simulink model "voltage_inverter"  (R2023a)
settings: Solver=VariableStepAuto  StartTime=0.0  StopTime=0.2  RelTol=1e-3
undefined symbols (not defined in the file): frequency, fsw, kpi, kpv, krv, omega, vc_c, vc_l, vdc, vref_rms
libraries: spsGroundLib x3, spsHalfBridgeConverterLib x3, spsThreePhaseParallelRLCBranchLib x3, spsThreePhaseVIMeasurementLib x3, spsabctoAlphaBetaZeroLib x3, spsAlphaBetaZerotoabcLib x1, spsDCVoltageSourceLib x1, eePwmGeneratorTwoLevel x1, spsThreePhaseProgrammableVoltageSourceLib x1, spspowerguiLib x1
settings Model: Creator=MrSam  LastModifiedBy=15185

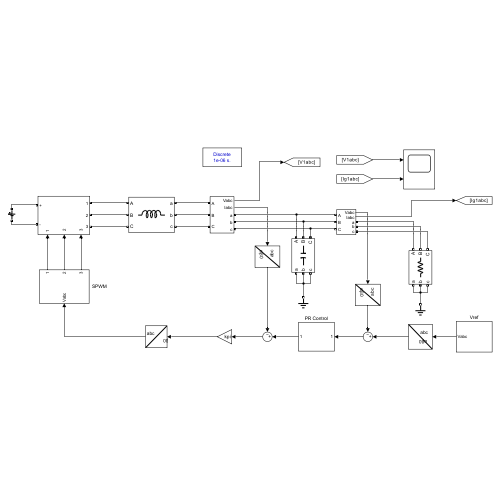
[thumbnail: Simulink's stored preview of the top-level diagram]
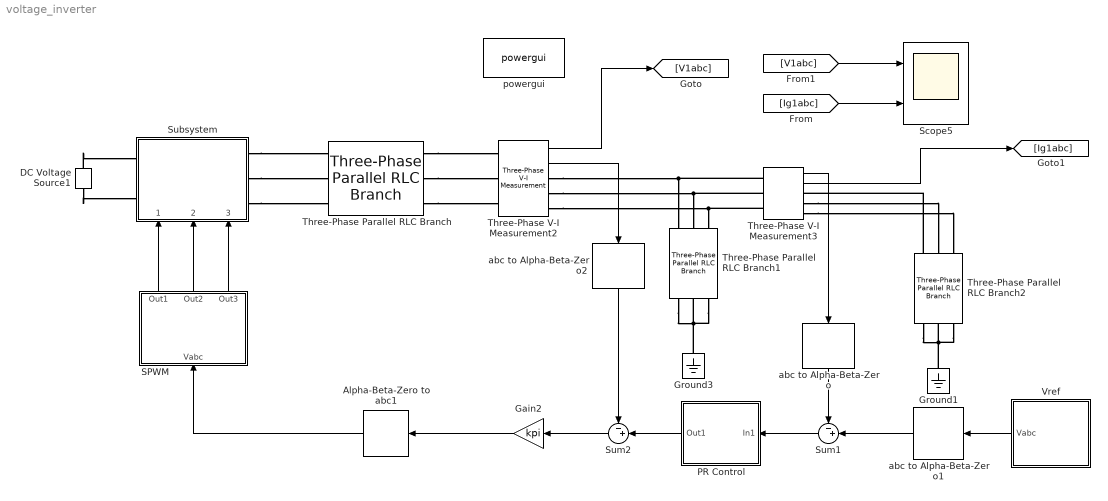
== system voltage_inverter ==
  Alpha-Beta-Zero to abc1 : spsAlphaBetaZerotoabcLib/Alpha-Beta-Zero to abc
      settings: LibrarySourceBlock=|
      | sps_lib/Control/Alpha-Beta-Zero
      | to abc
  DC Voltage Source1 : spsDCVoltageSourceLib/DC Voltage Source  Amplitude=vdc  Measurements=None
  Gain2 : Gain  Gain=kpi
  Ground1 : spsGroundLib/Ground  LConnTagsString=a
  Ground3 : spsGroundLib/Ground  LConnTagsString=a
  PR Control : Subsystem
  SPWM : Subsystem
  Scope5 : Scope  NumInputPorts=2
  Subsystem : Subsystem
      settings: PortSchema="{\"entries\":[{\"content\":{\"sides\":[{\"content\":{\"connectorIds\":[\"LConn1\",\"LConn2\"]},\"type\":\"ConnectorPlacement.EquallySpacedRectSide\",\"uuid\":\"21765539-0567-4900-b052-fb0c809e49e6\"},{\"content\":{\"connectorIds\":[\"RConn1\",\"RConn2\",\"RConn3\"],\"side\":\"RIGHT\"},\"type\":\"ConnectorPlacement.EquallySpacedRectSide\",\"uuid\":\"da60e673-aefd-4ef6-b5b1-e42a137712f7\"},{\"content\":{\"side\":\"TOP\"},\"type\":\"ConnectorPlacement.EquallySpacedRectSide\",\"uuid\":\"b6e664be-1a8c-4c9c-bd73-b93bd6e53381\"},{\"content\":{\"connectorIds\":[\"In1\",\"In2\",\"In3\"],\"side\":\"BOTTOM\"},\"type\":\"ConnectorPlacement.EquallySpacedRectSide\",\"uuid\":\"f785bed7-33ce-41e0-9620-ddd9724794f7\"}]},\"type\":\"ConnectorPlacement.EquallySpacedConnector\",\"uuid\":\"3eaff965-cae1-44ee-8f3f-ae8df46f200b\"}],\"packageUris\":[\"http://schema.mathworks.com/mf0/Connector/R2020b\"],\"version\":\"1.0\"}"
  Sum1 : Sum  Inputs=-+|
  Sum2 : Sum  Inputs=-+|
  Three-Phase Parallel RLC Branch : spsThreePhaseParallelRLCBranchLib/Three-Phase Parallel RLC Branch  LConnTagsString=A|B|C  RConnTagsString=A|B|C  BranchType=L  Resistance=1  Inductance=vc_l/(2*pi*frequency)  Capacitance=1e-6  Measurements=None
  Three-Phase Parallel RLC Branch1 : spsThreePhaseParallelRLCBranchLib/Three-Phase Parallel RLC Branch  LConnTagsString=A|B|C  RConnTagsString=A|B|C  BranchType=C  Resistance=1  Inductance=vc_l  Capacitance=1/(vc_c*2*pi*frequency)  Measurements=None
  Three-Phase Parallel RLC Branch2 : spsThreePhaseParallelRLCBranchLib/Three-Phase Parallel RLC Branch  LConnTagsString=A|B|C  RConnTagsString=A|B|C  BranchType=R  Resistance=10  Inductance=1e-3  Capacitance=1e-6  Measurements=None
  Three-Phase V-I Measurement2 : spsThreePhaseVIMeasurementLib/Three-Phase V-I Measurement  VoltageMeasurement=phase-to-ground  SetLabelV=off  LabelV=Vabc  Vpu=off  VpuLL=off  CurrentMeasurement=yes  SetLabelI=off  LabelI=Iabc  Ipu=off  Pbase=100e6  Vbase=500e3  OutputType=Complex  PhasorSimulation=off  PSBequivalent=0
  Three-Phase V-I Measurement3 : spsThreePhaseVIMeasurementLib/Three-Phase V-I Measurement  VoltageMeasurement=phase-to-ground  SetLabelV=off  LabelV=Vabc  Vpu=off  VpuLL=off  CurrentMeasurement=yes  SetLabelI=off  LabelI=Iabc  Ipu=off  Pbase=100e6  Vbase=500e3  OutputType=Complex  PhasorSimulation=off  PSBequivalent=0
  Vref : Subsystem
  abc to Alpha-Beta-Zero : spsabctoAlphaBetaZeroLib/abc to Alpha-Beta-Zero
  abc to Alpha-Beta-Zero1 : spsabctoAlphaBetaZeroLib/abc to Alpha-Beta-Zero
  abc to Alpha-Beta-Zero2 : spsabctoAlphaBetaZeroLib/abc to Alpha-Beta-Zero
  powergui : spspowerguiLib/powergui  Priority=1  SimulationMode=Discrete  SampleTime=1e-6  frequency=60  Iterations=50  frequencyindice=50  Pbase=100e6  ErrMax=1e-4  UnitsV=kV  UnitsW=MW  buscounter=0  FunctionMessages=off  echomessages=off  EnableUseOfTLC=off  CurrentSourceSwitches=off  DisableSnubberDevices=off  DisableRonSwitches=off  DisableVfSwitches=off  DisplayEquations=off  AutomaticDiscreteSolvers=off  SolverType=Tustin/Backward Euler (TBE)  Interpol=off  ExternalGateDelay=off  methode=off  Ts=100  x0status=blocks  SPID=on  SwTol=0  HookPort=off  NonlinearTolerance=1e-4  nMaxIteration=100  ContinueOnMaxIteration=off  RestoreLinks=warning  ResistiveCurrentMeasurement=off  Frange=[0:2:500]  Ylog=off  Xlog=on  ShowGrid=off  save=off  variable=ZData  structure=0  ZoomFFT=off  StartTime=0.0  cycles=1  DisplayStyle=1  fundamental=60  FreqAxis=off  MaxFrequency=1000  frequencyindicesteady=1  RmsSteady=1  display=off
  wires:
  Three-Phase V-I Measurement3/1 -> abc to Alpha-Beta-Zero/1
  abc to Alpha-Beta-Zero1/1 -> Sum1/2
  abc to Alpha-Beta-Zero/1 -> Sum1/1
  abc to Alpha-Beta-Zero2/1 -> Sum2/1
  Three-Phase V-I Measurement2/2 -> abc to Alpha-Beta-Zero2/1
  Sum2/1 -> Gain2/1
  Gain2/1 -> Alpha-Beta-Zero to abc1/1
  Sum1/1 -> PR Control/1(In1)
  PR Control/1(Out1) -> Sum2/2
  Vref/1(Vabc) -> abc to Alpha-Beta-Zero1/1
  Alpha-Beta-Zero to abc1/1 -> SPWM/1(Vabc)
  SPWM/1(Out1) -> Subsystem/1(" 1 ")
  SPWM/2(Out2) -> Subsystem/2("  2")
  SPWM/3(Out3) -> Subsystem/3("  3")
  Three-Phase V-I Measurement2/1 -> [V1abc]
  [Ig1abc] -> Scope5/2
  [V1abc] -> Scope5/1
  Three-Phase V-I Measurement3/2 -> [Ig1abc]
  connections:
  Three-Phase Parallel RLC Branch/RConn1 -- Three-Phase V-I Measurement2/LConn1
  Three-Phase Parallel RLC Branch/RConn2 -- Three-Phase V-I Measurement2/LConn2
  Three-Phase Parallel RLC Branch/RConn3 -- Three-Phase V-I Measurement2/LConn3
  Three-Phase V-I Measurement2/RConn1 -- Three-Phase Parallel RLC Branch1/LConn1 -- Three-Phase V-I Measurement3/LConn1
  Three-Phase V-I Measurement2/RConn2 -- Three-Phase V-I Measurement3/LConn2 -- Three-Phase Parallel RLC Branch1/LConn2
  Three-Phase V-I Measurement2/RConn3 -- Three-Phase Parallel RLC Branch1/LConn3 -- Three-Phase V-I Measurement3/LConn3
  Ground3/LConn1 -- Three-Phase Parallel RLC Branch1/RConn1 -- Three-Phase Parallel RLC Branch1/RConn3 -- Three-Phase Parallel RLC Branch1/RConn2
  Ground1/LConn1 -- Three-Phase Parallel RLC Branch2/RConn1 -- Three-Phase Parallel RLC Branch2/RConn3 -- Three-Phase Parallel RLC Branch2/RConn2
  DC Voltage Source1/RConn1 -- Subsystem/LConn1
  DC Voltage Source1/LConn1 -- Subsystem/LConn2
  Subsystem/RConn1 -- Three-Phase Parallel RLC Branch/LConn1
  Subsystem/RConn2 -- Three-Phase Parallel RLC Branch/LConn2
  Subsystem/RConn3 -- Three-Phase Parallel RLC Branch/LConn3
  Three-Phase V-I Measurement3/RConn3 -- Three-Phase Parallel RLC Branch2/LConn3
  Three-Phase Parallel RLC Branch2/LConn1 -- Three-Phase V-I Measurement3/RConn1
  Three-Phase V-I Measurement3/RConn2 -- Three-Phase Parallel RLC Branch2/LConn2

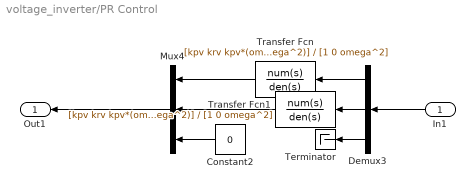
== system voltage_inverter/PR Control ==
  In1 : Inport
  Constant2 : Constant  Value=0
  Demux3 : Demux  Outputs=3
  Mux4 : Mux  Inputs=3
  Terminator : Terminator
  Transfer Fcn : TransferFcn  Numerator=[kpv krv kpv*(omega^2)]  Denominator=[1 0 omega^2]
  Transfer Fcn1 : TransferFcn  Numerator=[kpv krv kpv*(omega^2)]  Denominator=[1 0 omega^2]
  Out1 : Outport
  wires:
  Transfer Fcn/1 -> Mux4/1
  Mux4/1 -> Out1/1
  Demux3/1 -> Transfer Fcn/1
  Demux3/2 -> Transfer Fcn1/1
  Constant2/1 -> Mux4/3
  Transfer Fcn1/1 -> Mux4/2
  In1/1 -> Demux3/1
  Demux3/3 -> Terminator/1

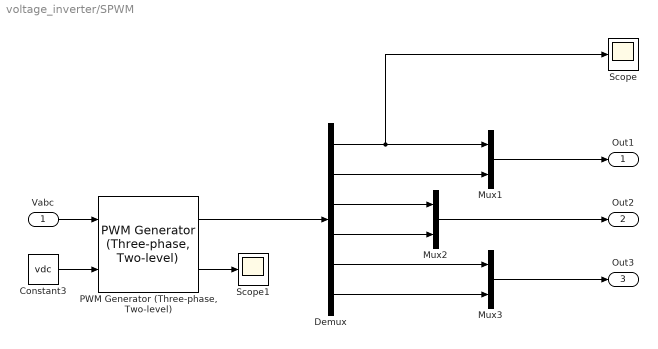
== system voltage_inverter/SPWM ==
  Vabc : Inport
  Constant3 : Constant  Value=vdc
  Demux : Demux  Outputs=6
  Mux1 : Mux  Inputs=2
  Mux2 : Mux  Inputs=2
  Mux3 : Mux  Inputs=2
  "PWM Generator (Three-phase, Two-level)" : eePwmGeneratorTwoLevel/PWM Generator (Three-phase, Two-level)  PWMMode=Continuous PWM (CPWM)  CPWMMode=SPWM: sinusoidal PWM  DPWMMode=60 DPWM: 60 degree discontinuous PWM  fsw=fsw  Ts=1/(60*fsw)
      settings: LibrarySourceBlock=|
      | ee_sl_lib/Pulse Width
      | Modulation/PWM Generator
      | (Three-phase, Two-level)
  Scope : Scope
  Scope1 : Scope
  Out1 : Outport
  Out2 : Outport  Port=2
  Out3 : Outport  Port=3
  wires:
  "PWM Generator (Three-phase, Two-level)"/2 -> Scope1/1
  Demux/2 -> Mux1/2
  Vabc/1 -> "PWM Generator (Three-phase, Two-level)"/1
  Demux/6 -> Mux3/2
  Demux/1 -> Scope/1, Mux1/1
  Constant3/1 -> "PWM Generator (Three-phase, Two-level)"/2
  Mux2/1 -> Out2/1
  Demux/4 -> Mux2/2
  "PWM Generator (Three-phase, Two-level)"/1 -> Demux/1
  Demux/3 -> Mux2/1
  Demux/5 -> Mux3/1
  Mux1/1 -> Out1/1
  Mux3/1 -> Out3/1

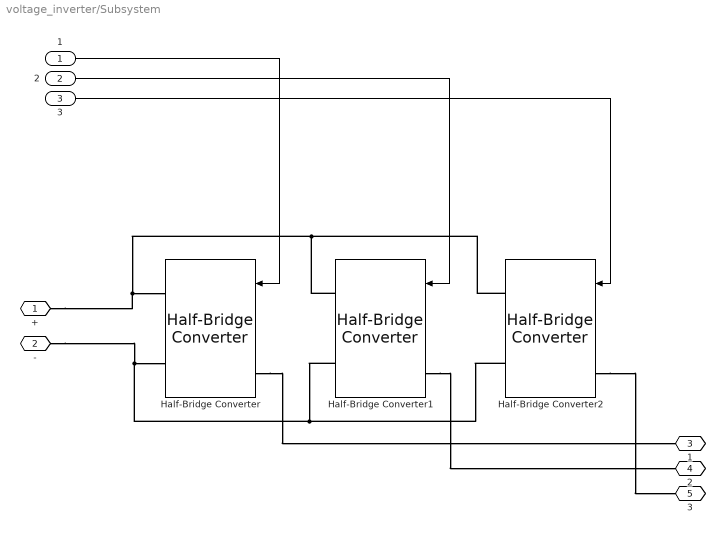
== system voltage_inverter/Subsystem ==
  " 1 " : Inport
  "  2" : Inport  Port=2
  "  3" : Inport  Port=3
  Half-Bridge Converter : spsHalfBridgeConverterLib/Half-Bridge Converter  ModelType=Switching devices  Ron=1e-3  Rs=1e6  Cs=inf  Vforward=[0,0]  Ron_Diode=1e-3  Rs_Diode=1e6  Cs_Diode=inf  Vf_Diode=1e-3  Rs_CurrentSource=inf  Ron_ACsource=1e-3
      settings: LibrarySourceBlock=sps_lib/Power Electronics/Half-Bridge Converter
  Half-Bridge Converter1 : spsHalfBridgeConverterLib/Half-Bridge Converter  ModelType=Switching devices  Ron=1e-3  Rs=1e6  Cs=inf  Vforward=[0,0]  Ron_Diode=1e-3  Rs_Diode=1e6  Cs_Diode=inf  Vf_Diode=1e-3  Rs_CurrentSource=inf  Ron_ACsource=1e-3
      settings: LibrarySourceBlock=sps_lib/Power Electronics/Half-Bridge Converter
  Half-Bridge Converter2 : spsHalfBridgeConverterLib/Half-Bridge Converter  ModelType=Switching devices  Ron=1e-3  Rs=1e6  Cs=inf  Vforward=[0,0]  Ron_Diode=1e-3  Rs_Diode=1e6  Cs_Diode=inf  Vf_Diode=1e-3  Rs_CurrentSource=inf  Ron_ACsource=1e-3
      settings: LibrarySourceBlock=sps_lib/Power Electronics/Half-Bridge Converter
  + : PMIOPort  Side=Left
  - : PMIOPort  Port=2  Side=Left
  1 : PMIOPort  Port=3  Side=Right
  2 : PMIOPort  Port=4  Side=Right
  3 : PMIOPort  Port=5  Side=Right
  wires:
  "  2"/1 -> Half-Bridge Converter1/1
  "  3"/1 -> Half-Bridge Converter2/1
  " 1 "/1 -> Half-Bridge Converter/1
  connections:
  Half-Bridge Converter/LConn1 -- 1/RConn1
  Half-Bridge Converter1/RConn1 -- Half-Bridge Converter2/RConn1 -- +/RConn1 -- Half-Bridge Converter/RConn1
  Half-Bridge Converter2/RConn2 -- Half-Bridge Converter1/RConn2 -- -/RConn1 -- Half-Bridge Converter/RConn2
  Half-Bridge Converter2/LConn1 -- 3/RConn1
  Half-Bridge Converter1/LConn1 -- 2/RConn1

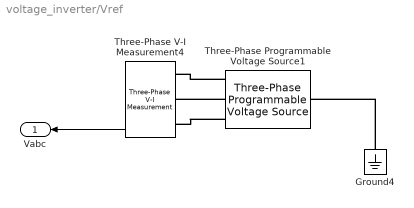
== system voltage_inverter/Vref ==
  Ground4 : spsGroundLib/Ground  LConnTagsString=a
  Three-Phase Programmable Voltage Source1 : spsThreePhaseProgrammableVoltageSourceLib/Three-Phase Programmable Voltage Source  PositiveSequence="[vref_rms  0 frequency]"  VariationEntity=None  VariationType=Table of time-amplitude pairs  VariationTypeAlt=Step  VariationStep=0.5  VariationRate=10  VariationMagnitude=0.3  VariationFrequency=2  VariationTiming=[1 2]  VariationPhaseA=off  Amplitudes=[1 0.8 1.2 1.0]  TimeValues=[0 0.1 0.15 0.2]  HarmonicGeneration=off  HarmonicA=[3 0.2 -25 0]  HarmonicB=[2 0.15 35 2]  Timing="[0.05  3]"  BusType=swing  Pref=0  Qref=0  Qmin=-inf  Qmax=inf
  Three-Phase V-I Measurement4 : spsThreePhaseVIMeasurementLib/Three-Phase V-I Measurement  VoltageMeasurement=phase-to-ground  SetLabelV=off  LabelV=Vabc  Vpu=off  VpuLL=off  CurrentMeasurement=yes  SetLabelI=off  LabelI=Iabc  Ipu=off  Pbase=100e6  Vbase=500e3  OutputType=Complex  PhasorSimulation=off  PSBequivalent=0
  Vabc : Outport
  wires:
  Three-Phase V-I Measurement4/1 -> Vabc/1
  connections:
  Three-Phase Programmable Voltage Source1/RConn2 -- Three-Phase V-I Measurement4/LConn2
  Three-Phase Programmable Voltage Source1/RConn3 -- Three-Phase V-I Measurement4/LConn3
  Three-Phase Programmable Voltage Source1/RConn1 -- Three-Phase V-I Measurement4/LConn1
  Ground4/LConn1 -- Three-Phase Programmable Voltage Source1/LConn1
